simulink model "StateMachine_v3"  (R2015a)
settings: Solver=ode1  StartTime=0.0  StopTime=Inf  FixedStep=0.001  RelTol=1e-3
PreLoadFcn:
  | LoadVar
PostLoadFcn:
  | , if any(exist('dsrtsu_mdlpostloadfcn', 'file') == [2, 3, 6]), try dsrtsu_mdlpostloadfcn('Execute', bdroot); catch fprintf('Error in PostLoadFcn (dsrtsu_mdlpostloadfcn) for model "%s":\n %s\n', bdroot, lasterr); end, end,
values from neighbouring files (symbols this model uses):
  AllowReset = 0    [LoadVar.m]
  Brake_Limits = [Brake_lowerlim1,Brake_upperlim1,Brake_lowerlim2,Brake_upperlim2]    [LoadVar.m]
  DcCLimGen = 0    [LoadVar.m]
  DcCLimMot = 20    [LoadVar.m]
  DcVLimGen = 400    [LoadVar.m]
  DcVLimMot = 280    [LoadVar.m]
  DifferentialFactor = 0.5    [LoadVar.m]
  MaxDisplacementSteeringRack = 21.08    [LoadVar.m]
  MaxSteeringAngle = 24.635    [LoadVar.m]
  MechPwrMaxGen = 3000    [LoadVar.m]
  MechPwrMaxMot = 3000    [LoadVar.m]
  PowerLim_W = 3000    [LoadVar.m]
  SpdSlewrate = 1000    [LoadVar.m]
  Steer_Limits = [Steer_lowerlim,Steer_upperlim,Steer_zero]    [LoadVar.m]
  Susp_Limits = [Susp_lowerlim1,Susp_upperlim1,Susp_lowerlim2,Susp_upperlim2,Susp_lowerlim3,Susp_upperlim3,Susp_lowerlim4,Susp_upperlim4]    [LoadVar.m]
  Throttle_Limits = [Throttle_lowerlim1,Throttle_upperlim1,Throttle_lowerlim2,Throttle_upperlim2]    [LoadVar.m]
  TrqSlewrate = 3    [LoadVar.m]
libraries: rtican x25, rti1401lib_adc_type4 x16, rti1401lib_dio_type3 x16, rtilib1401 x1
(part 7 of 7)

== system StateMachine_v3/PRE-PROCESSOR/SteeringAngleCalculation ==
  SteeringAngleTravel_% : Inport
  limits : Inport  Port=2
  1-D Lookup Table : Lookup_n-D  NumberOfTableDimensions=1  BreakpointsForDimension1=[-MaxDisplacementSteeringRack,-20.1,-19.12,-18.14,-17.15,-16.18,-15.2,-14.22,-13.25,-12.27,-11.3,-10.34,-9.38,-8.42,-7.46,-6.51,-5.56,-4.62,-3.69,-2.75,-1.83,-0.91,0,0.91,1.83,2.75,3.69,4.62,5.56,6.51,7.46,8.42,9.38,10.34,11.3,12.27,13.25,14.22,15.2,16.18,17.15,18.14,19.12,20.1,MaxDisplacementSteeringRack]  Table=[-MaxSteeringAngle,-23.33,-22.06,-20.81,-19.59,-18.385,-17.205,-16.035,-14.855,-13.75,-12.63,-11.52,-10.425,-9.34,-8.265,-7.2,-6.145,-5.1,-4.065,-3.035,-2.015,-1.05,0,1.05,2.015,3.035,4.065,5.1,6.145,7.2,8.265,9.34,10.425,11.52,12.63,13.75,14.855,16.035,17.205,18.385,19.59,20.81,22.06,23.33,MaxSteeringAngle]  InternalRulePriority=Speed  RndMeth=Simplest  InputSameDT=on
  Constant : Constant  Value=MaxDisplacementSteeringRack
  MATLAB Function : MATLAB Function  TreatAsAtomicUnit=on
  SteeringAngle_° : Outport
  SteeringAngleSensorError : Outport  Port=2
  wires:
  MATLAB Function/2(e) -> SteeringAngleSensorError/1
  limits/1 -> MATLAB Function/3(limits)
  MATLAB Function/1(SteeringDisplacement) -> 1-D Lookup Table/1  "SteeringDisplacement_mm"
  SteeringAngleTravel_%/1 -> MATLAB Function/1(SteeringAngleTravel)
  1-D Lookup Table/1 -> SteeringAngle_°/1  "SteeringAngle_°"
  Constant/1 -> MATLAB Function/2(MaxDisplacementSteeringRack)

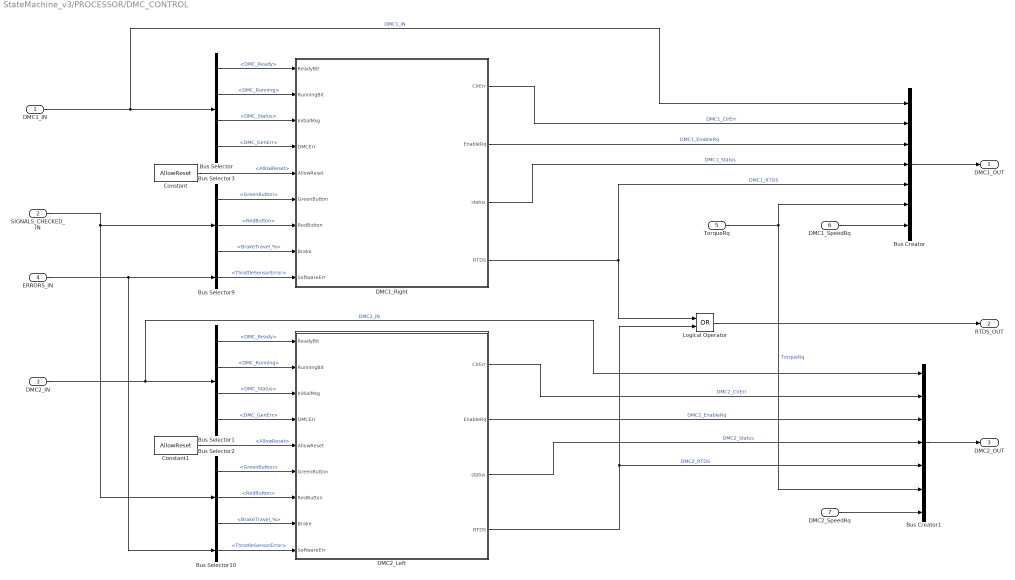
== system StateMachine_v3/PROCESSOR/DMC_CONTROL ==
  DMC1_IN : Inport
  SIGNALS_CHECKED_IN : Inport  Port=2
  DMC2_IN : Inport  Port=3
  ERRORS_IN : Inport  Port=4
  TorqueRq : Inport  Port=5
  DMC1_SpeedRq : Inport  Port=6
  DMC2_SpeedRq : Inport  Port=7
  Bus Creator : BusCreator  Inputs=7
  Bus Creator1 : BusCreator  Inputs=7
  Bus Selector : BusSelector  OutputSignals=DMC_Ready,DMC_Running,DMC_Status,DMC_GenErr
  Bus Selector1 : BusSelector  OutputSignals=DMC_Ready,DMC_Running,DMC_Status,DMC_GenErr
  Bus Selector10 : BusSelector  OutputSignals=ThrottleSensorError
  Bus Selector2 : BusSelector  OutputSignals=SIGNALS.DigitalInputs.GreenButton,SIGNALS.DigitalInputs.RedButton,BrakeTravel_%
  Bus Selector3 : BusSelector  OutputSignals=SIGNALS.DigitalInputs.GreenButton,SIGNALS.DigitalInputs.RedButton,BrakeTravel_%
  Bus Selector9 : BusSelector  OutputSignals=ThrottleSensorError
  Constant : Constant  Value=AllowReset
  Constant1 : Constant  Value=AllowReset
  DMC1_Right : Stateflow chart  TreatAsAtomicUnit=on
  DMC2_Left : Stateflow chart  TreatAsAtomicUnit=on
  Logical Operator : Logic  Operator=OR  AllPortsSameDT=off  OutDataTypeStr=boolean
  DMC1_OUT : Outport
  RTDS_OUT : Outport  Port=2
  DMC2_OUT : Outport  Port=3
  wires:
  TorqueRq/1 -> Bus Creator1/6, Bus Creator/6  "TorqueRq"
  ERRORS_IN/1 -> Bus Selector10/1, Bus Selector9/1
  SIGNALS_CHECKED_IN/1 -> Bus Selector2/1, Bus Selector3/1
  DMC1_Right/3(status) -> Bus Creator/4  "DMC1_Status"
  Bus Creator/1 -> DMC1_OUT/1
  Bus Selector9/1 -> DMC1_Right/9(SoftwareErr)  "<ThrottleSensorError>"
  Bus Selector10/1 -> DMC2_Left/9(SoftwareErr)  "<ThrottleSensorError>"
  Bus Creator1/1 -> DMC2_OUT/1
  Bus Selector/4 -> DMC1_Right/4(DMCErr)  "<DMC_GenErr>"
  Bus Selector3/2 -> DMC1_Right/7(RedButton)  "<RedButton>"
  DMC2_IN/1 -> Bus Creator1/1, Bus Selector1/1  "DMC2_IN"
  Bus Selector1/4 -> DMC2_Left/4(DMCErr)  "<DMC_GenErr>"
  DMC1_SpeedRq/1 -> Bus Creator/7
  DMC2_Left/3(status) -> Bus Creator1/4  "DMC2_Status"
  Bus Selector2/3 -> DMC2_Left/8(Brake)  "<BrakeTravel_%>"
  DMC2_Left/4(RTDS) -> Bus Creator1/5, Logical Operator/2  "DMC2_RTDS"
  DMC1_Right/4(RTDS) -> Logical Operator/1, Bus Creator/5  "DMC1_RTDS"
  Logical Operator/1 -> RTDS_OUT/1
  DMC2_Left/1(ClrErr) -> Bus Creator1/2  "DMC2_ClrErr"
  Constant1/1 -> DMC2_Left/5(AllowReset)  "<AllowReset>"
  Bus Selector1/2 -> DMC2_Left/2(RunningBit)  "<DMC_Running>"
  DMC1_IN/1 -> Bus Creator/1, Bus Selector/1  "DMC1_IN"
  DMC1_Right/1(ClrErr) -> Bus Creator/2  "DMC1_ClrErr"
  DMC2_SpeedRq/1 -> Bus Creator1/7
  Bus Selector1/1 -> DMC2_Left/1(ReadyBit)  "<DMC_Ready>"
  Bus Selector3/1 -> DMC1_Right/6(GreenButton)  "<GreenButton>"
  Bus Selector/3 -> DMC1_Right/3(InitialMsg)  "<DMC_Status>"
  Bus Selector1/3 -> DMC2_Left/3(InitialMsg)  "<DMC_Status>"
  Bus Selector/1 -> DMC1_Right/1(ReadyBit)  "<DMC_Ready>"
  Bus Selector3/3 -> DMC1_Right/8(Brake)  "<BrakeTravel_%>"
  Bus Selector2/2 -> DMC2_Left/7(RedButton)  "<RedButton>"
  DMC2_Left/2(EnableRq) -> Bus Creator1/3  "DMC2_EnableRq"
  Bus Selector/2 -> DMC1_Right/2(RunningBit)  "<DMC_Running>"
  Bus Selector2/1 -> DMC2_Left/6(GreenButton)  "<GreenButton>"
  Constant/1 -> DMC1_Right/5(AllowReset)  "<AllowReset>"
  DMC1_Right/2(EnableRq) -> Bus Creator/3  "DMC1_EnableRq"

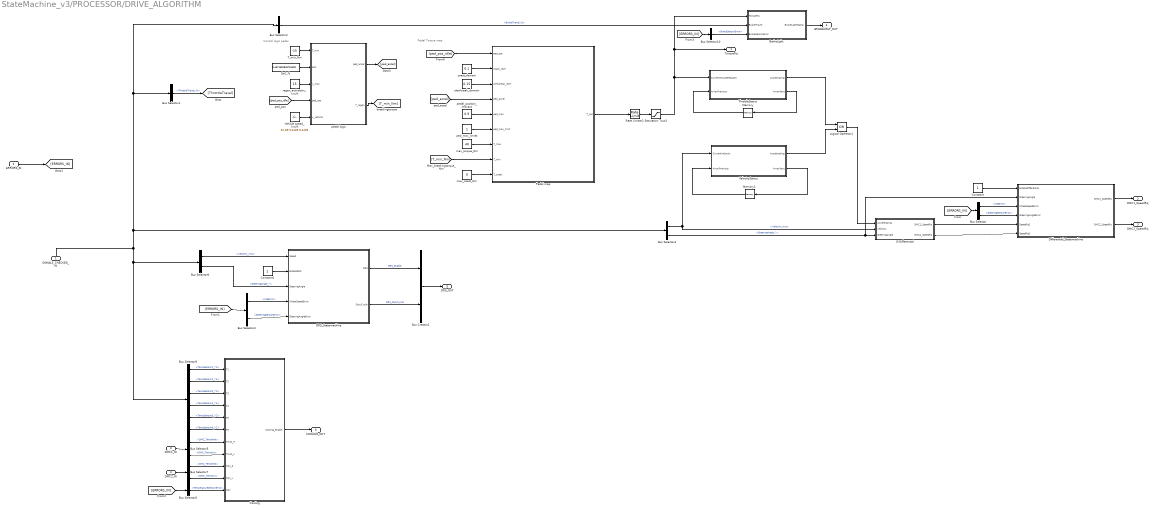
== system StateMachine_v3/PROCESSOR/DRIVE_ALGORITHM ==
  note: Control logic pedal
  note: Pedal Torque map
  SIGNALS_CHECKED_IN : Inport
  ERRORS_IN : Inport  Port=2
  DMC1_IN : Inport  Port=3
  DMC2_IN : Inport  Port=4
  BrakeLight : MATLAB Function  TreatAsAtomicUnit=on
  Bus Creator2 : BusCreator  Inputs=2
  Bus Selector : BusSelector  OutputSignals=WSError,SteeringSensorError
  Bus Selector1 : BusSelector  OutputSignals=ThrottleTravel_%
  Bus Selector10 : BusSelector  OutputSignals=BrakeSensorError
  Bus Selector2 : BusSelector  OutputSignals=BrakeTravel_%
  Bus Selector3 : BusSelector  OutputSignals=WSError,SteeringSensorError
  Bus Selector4 : BusSelector  OutputSignals=Velocity_m/s,SteeringAngle_°
  Bus Selector5 : BusSelector  OutputSignals=DMC_TempMot,DMC_TempInv
  Bus Selector6 : BusSelector  OutputSignals=TemperatureSensorError
  Bus Selector7 : BusSelector  OutputSignals=DMC_TempMot,DMC_TempInv
  Bus Selector8 : BusSelector  OutputSignals=Velocity_m/s,SteeringAngle_°
  Bus Selector9 : BusSelector  OutputSignals=TempSensor1_°C,TempSensor2_°C,TempSensor3_°C,TempSensor4_°C,TempSensor5_°C,TempSensor6_°C
  Constant : Constant
  Constant1 : Constant
  Cooling : MATLAB Function  TreatAsAtomicUnit=on
  DRS_Statemachine : Stateflow chart  TreatAsAtomicUnit=on
  Differential_Statemachine : Stateflow chart  TreatAsAtomicUnit=on
  E-Differential : Subsystem
  Logical Operator1 : Logic  Operator=OR  AllPortsSameDT=off  OutDataTypeStr=boolean
  Memory : Memory  X0=zeros(10,1)  InheritSampleTime=on
  Memory1 : Memory  X0=zeros(10,1)  InheritSampleTime=on
  Pedal map : MATLAB Function  TreatAsAtomicUnit=on
  Rate Limiter2 : RateLimiter  RisingSlewLimit=20  FallingSlewLimit=-20  SampleTimeMode=inherited
  Saturation Tout1 : Saturate  UpperLimit=39  LowerLimit=-39
  SoC_% : Constant  Value=0.4671532846715328
  T_min_Nm : Constant  Value=-15
  ThrottleStatus : MATLAB Function  TreatAsAtomicUnit=on
  Vehicle speed_km/h : Constant  Value=52.85714285714285
  VelocityStatus : MATLAB Function  TreatAsAtomicUnit=on
  coast_domain : Constant  Value=0.1
  max_coast_Nm : Constant  Value=0
  max_torque_Nm : Constant  Value=40
  ped_max_limiet : Constant
  pedal logic : Stateflow chart  TreatAsAtomicUnit=on
  pedal_position_maxacc : Constant  Value=0.9
  regen_activation_km/h : Constant  Value=15
  slewbreak_domain : Constant  Value=0.15
  TorqueRq : Outport
  DMC1_SpeedRq : Outport  Port=2
  DMC2_SpeedRq : Outport  Port=3
  BRAKELIGHT_OUT : Outport  Port=4
  DRS_OUT : Outport  Port=5
  COOLING_OUT : Outport  Port=6
  wires:
  Bus Selector1/1 -> [ThrottleTravel]  "<ThrottleTravel_%>"
  DRS_Statemachine/1(DRS) -> Bus Creator2/1  "DRS_Enable"
  DRS_Statemachine/2(DutyCycle) -> Bus Creator2/2  "DRS_DutyCycle"
  Bus Creator2/1 -> DRS_OUT/1
  Bus Selector8/2 -> DRS_Statemachine/3(SteeringAngle)  "<SteeringAngle_°>"
  Bus Selector8/1 -> DRS_Statemachine/1(Speed)  "<Velocity_m/s>"
  SIGNALS_CHECKED_IN/1 -> Bus Selector1/1, Bus Selector2/1, Bus Selector4/1, Bus Selector9/1, Bus Selector8/1
  Constant1/1 -> DRS_Statemachine/2(EnableDRS)
  Saturation Tout1/1 -> BrakeLight/1(TorqueRq), TorqueRq/1, ThrottleStatus/1(CurrentTorqueRequest)
  Pedal map/1(T_out) -> Rate Limiter2/1
  [ped_accel] -> Pedal map/4(ped_accel)
  Rate Limiter2/1 -> Saturation Tout1/1
  coast_domain/1 -> Pedal map/2(coast_dom)
  Vehicle speed_km/h/1 -> pedal logic/5(v_vehicle)
  [ped_pos_idle] -> pedal logic/4(ped_pos)
  pedal_position_maxacc/1 -> Pedal map/5(ped_max)
  T_min_Nm/1 -> pedal logic/1(T_min)
  ped_max_limiet/1 -> Pedal map/6(ped_max_limit)
  [ped_pos_idle] -> Pedal map/1(ped_pos)
  slewbreak_domain/1 -> Pedal map/3(slewbreak_dom)
  [T_min_Nm] -> Pedal map/8(T_min)
  SoC_%/1 -> pedal logic/2(SoC)
  pedal logic/2(T_regen) -> [T_min_Nm]
  max_torque_Nm/1 -> Pedal map/7(T_max)
  pedal logic/1(ped_accel) -> [ped_accel]
  regen_activation_km/h/1 -> pedal logic/3(v_max)
  max_coast_Nm/1 -> Pedal map/9(T_coast)
  Bus Selector4/2 -> Differential_Statemachine/2(SteeringAngle), E-Differential/3(SteeringAngle)  "<SteeringAngle_°>"
  Bus Selector4/1 -> VelocityStatus/1(CurrentVelocity), E-Differential/2(Velocity)  "<Velocity_m/s>"
  Bus Selector2/1 -> BrakeLight/2(BrakeTravel)  "<BrakeTravel_%>"
  BrakeLight/1(BrakeLightSignal) -> BRAKELIGHT_OUT/1
  Constant/1 -> Differential_Statemachine/1(EnableDifferential)
  Differential_Statemachine/2(DMC2_SpeedRq) -> DMC2_SpeedRq/1
  Differential_Statemachine/1(DMC1_SpeedRq) -> DMC1_SpeedRq/1
  E-Differential/1(DMC1_SpeedRq) -> Differential_Statemachine/5(SpeedRq1)
  E-Differential/2(DMC2_SpeedRq) -> Differential_Statemachine/6(SpeedRq2)
  Memory/1 -> ThrottleStatus/2(ArrayPrevious)
  ThrottleStatus/2(ArrayNext) -> Memory/1
  VelocityStatus/2(ArrayNext) -> Memory1/1
  Memory1/1 -> VelocityStatus/2(ArrayPrevious)
  ThrottleStatus/1(Accelerating) -> Logical Operator1/1
  VelocityStatus/1(Accelerating) -> Logical Operator1/2
  Logical Operator1/1 -> E-Differential/1(Accelerating)
  ERRORS_IN/1 -> [ERRORS_IN]
  [ERRORS_IN] -> Bus Selector/1
  Bus Selector/2 -> Differential_Statemachine/4(SteeringAngleError)  "<SteeringSensorError>"
  Bus Selector/1 -> Differential_Statemachine/3(WheelSpeedError)  "<WSError>"
  Bus Selector3/1 -> DRS_Statemachine/4(WheelSpeedError)  "<WSError>"
  Bus Selector3/2 -> DRS_Statemachine/5(SteeringAngleError)  "<SteeringSensorError>"
  [ERRORS_IN] -> Bus Selector3/1
  DMC1_IN/1 -> Bus Selector5/1
  DMC2_IN/1 -> Bus Selector7/1
  [ERRORS_IN] -> Bus Selector6/1
  Bus Selector9/1 -> Cooling/1(T1)  "<TempSensor1_°C>"
  Bus Selector9/2 -> Cooling/2(T2)  "<TempSensor2_°C>"
  Bus Selector6/1 -> Cooling/11(Terr)  "<TemperatureSensorError>"
  Bus Selector9/4 -> Cooling/4(T4)  "<TempSensor4_°C>"
  Bus Selector9/6 -> Cooling/6(T6)  "<TempSensor6_°C>"
  Bus Selector9/5 -> Cooling/5(T5)  "<TempSensor5_°C>"
  Bus Selector9/3 -> Cooling/3(T3)  "<TempSensor3_°C>"
  Bus Selector5/1 -> Cooling/7(Tmot_R)  "<DMC_TempMot>"
  Bus Selector5/2 -> Cooling/8(Tmot_L)  "<DMC_TempInv>"
  Bus Selector7/1 -> Cooling/9(Tdri_R)  "<DMC_TempMot>"
  Bus Selector7/2 -> Cooling/10(Tdri_L)  "<DMC_TempInv>"
  Cooling/1(Cooling_Enable) -> COOLING_OUT/1
  [ERRORS_IN] -> Bus Selector10/1
  Bus Selector10/1 -> BrakeLight/3(BrakeSensorError)  "<BrakeSensorError>"

== system StateMachine_v3/RTI Data/RTI Data Store ==
  RTI Data Store : Subsystem  mask(RTI_DATA_STORE){}
      mask help:
      | RTI Data Store Block. This block is used by RTI to store internal model dependent data. Deleting this block will result in data loss.
      |
      | NEVER DELETE, COPY, OR MODIFY THIS BLOCK!
      mask Help:
      | RTI Data Store Block. This block is used by RTI to store internal model dependent data. Deleting this block will result in data loss.
      | 
      | NEVER DELETE, COPY, OR MODIFY THIS BLOCK!
      mask Display: text(0.5, 0.5, ' ', 'HorizontalAlignment', 'center');

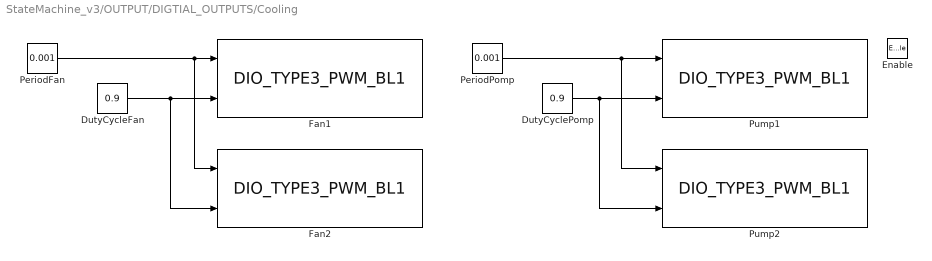
== system StateMachine_v3/OUTPUT/DIGTIAL_OUTPUTS/Cooling ==
  Enable : EnablePort
  DutyCycleFan : Constant  Value=0.9
  DutyCyclePomp : Constant  Value=0.9
  Fan1 : rti1401lib_dio_type3/DIO_TYPE3_PWM_BL1  DSProperties=struct('RTI',struct('Version',uint32(2),'BlockType',struct('isSLSource',uint8(0),'isSLSink',uint8(1),'isHWSource',uint8(0),'isHWSink',uint8(1),'isSetup',uint8(0),'isInline',uint8(1),'isNonInline',uint8(0),'isInterrupt',uint8(0),'isChannelwise',uint8(1)),'IOBoardType',{{'DS1401','STD','DIOT3'}},'UnitType','PWM','Identifier','PWM','DialogType','ML','BlockSet','NONE','SlaveProcessor','NONE'))  RTIBlockInterface=struct('InputPortsWidth',int32([1 1]),'InputPortsActive',[1 1],'InputPortsName',{{'Period',['Duty Cycle']}},'BlockDisplay',{{['DIO TP3 PWM\nModule: 1\nPort: 1\nChannel: 3'],'center'}},'IconTransparency','on','InitLevel',3,'DialogFcn','rti1401stddiot3pwmgui','BlockName',struct('Token',{{'DIO_TYPE3_PWM_BL1'}}))  RTIBlockParameters=struct('ModuleNo',{{1,'OFF',[1 16]}},'PortNo',{{1,'OFF',[1 3]}},'ChannelNo',{{3,'OFF',[1 16]}},'SupplyRailsCh',{{[1 1],'OFF',[0 1 0 1]}},'UpdateMode',{{1,'ON',[1 2]}},'PeriodRange',{{7,'OFF',[1 16]}},'DutyCycleInit',{{'0','OFF',[0 1]}},'PeriodInit',{{'5e-05','OFF',[]}},'TerminationMode',{{0,'OFF',[0 1]}},'OutputTermValidate',{{0,'OFF',[0 1]}},'OutputTermBuildCheck',{{0,'OFF',[]}},'DutyCycleTerm',{{'0','OFF',[0 1]}},'PeriodTerm',{{'5e-05','OFF',[]}},'TLCFileName',{{'rti1401dio_t3_pwm','OFF',[]}},'EnableInterrupt',{{0,'OFF',[0 1]}},'TriggerEdgeType',{{1,'OFF',[1 3]}})  RTISFcnParameters=struct('ModuleNo','int32','PortNo','int16','ChannelNo','int16','SupplyRailsCh','int16','UpdateMode','int16','PeriodRange','int16','DutyCycleInit','double','PeriodInit','double','TerminationMode','int16','OutputTermValidate','int16','DutyCycleTerm','double','PeriodTerm','double','TLCFileName','char','EnableInterrupt','int16','TriggerEdgeType','int32')  RTIBlockParaDefault=struct('ModuleNo',1,'PortNo',1,'ChannelNo',1,'SupplyRailsCh',[1 1],'UpdateMode',1,'PeriodRange',7,'DutyCycleInit',0,'PeriodInit',5e-05,'TerminationMode',0,'OutputTermValidate',0,'OutputTermBuildCheck',0,'DutyCycleTerm',0,'PeriodTerm',5e-05,'TLCFileName','rti1401dio_t3_pwm','EnableInterrupt',0,'TriggerEdgeType',1)
  Fan2 : rti1401lib_dio_type3/DIO_TYPE3_PWM_BL1  DSProperties=struct('RTI',struct('Version',uint32(2),'BlockType',struct('isSLSource',uint8(0),'isSLSink',uint8(1),'isHWSource',uint8(0),'isHWSink',uint8(1),'isSetup',uint8(0),'isInline',uint8(1),'isNonInline',uint8(0),'isInterrupt',uint8(0),'isChannelwise',uint8(1)),'IOBoardType',{{'DS1401','STD','DIOT3'}},'UnitType','PWM','Identifier','PWM','DialogType','ML','BlockSet','NONE','SlaveProcessor','NONE'))  RTIBlockInterface=struct('InputPortsWidth',int32([1 1]),'InputPortsActive',[1 1],'InputPortsName',{{'Period',['Duty Cycle']}},'BlockDisplay',{{['DIO TP3 PWM\nModule: 1\nPort: 1\nChannel: 4'],'center'}},'IconTransparency','on','InitLevel',3,'DialogFcn','rti1401stddiot3pwmgui','BlockName',struct('Token',{{'DIO_TYPE3_PWM_BL1'}}))  RTIBlockParameters=struct('ModuleNo',{{1,'OFF',[1 16]}},'PortNo',{{1,'OFF',[1 3]}},'ChannelNo',{{4,'OFF',[1 16]}},'SupplyRailsCh',{{[1 1],'OFF',[0 1 0 1]}},'UpdateMode',{{1,'ON',[1 2]}},'PeriodRange',{{7,'OFF',[1 16]}},'DutyCycleInit',{{'0','OFF',[0 1]}},'PeriodInit',{{'5e-05','OFF',[]}},'TerminationMode',{{0,'OFF',[0 1]}},'OutputTermValidate',{{0,'OFF',[0 1]}},'OutputTermBuildCheck',{{0,'OFF',[]}},'DutyCycleTerm',{{'0','OFF',[0 1]}},'PeriodTerm',{{'5e-05','OFF',[]}},'TLCFileName',{{'rti1401dio_t3_pwm','OFF',[]}},'EnableInterrupt',{{0,'OFF',[0 1]}},'TriggerEdgeType',{{1,'OFF',[1 3]}})  RTISFcnParameters=struct('ModuleNo','int32','PortNo','int16','ChannelNo','int16','SupplyRailsCh','int16','UpdateMode','int16','PeriodRange','int16','DutyCycleInit','double','PeriodInit','double','TerminationMode','int16','OutputTermValidate','int16','DutyCycleTerm','double','PeriodTerm','double','TLCFileName','char','EnableInterrupt','int16','TriggerEdgeType','int32')  RTIBlockParaDefault=struct('ModuleNo',1,'PortNo',1,'ChannelNo',1,'SupplyRailsCh',[1 1],'UpdateMode',1,'PeriodRange',7,'DutyCycleInit',0,'PeriodInit',5e-05,'TerminationMode',0,'OutputTermValidate',0,'OutputTermBuildCheck',0,'DutyCycleTerm',0,'PeriodTerm',5e-05,'TLCFileName','rti1401dio_t3_pwm','EnableInterrupt',0,'TriggerEdgeType',1)
  PeriodFan : Constant  Value=0.001
  PeriodPomp : Constant  Value=0.001
  Pump1 : rti1401lib_dio_type3/DIO_TYPE3_PWM_BL1  DSProperties=struct('RTI',struct('Version',uint32(2),'BlockType',struct('isSLSource',uint8(0),'isSLSink',uint8(1),'isHWSource',uint8(0),'isHWSink',uint8(1),'isSetup',uint8(0),'isInline',uint8(1),'isNonInline',uint8(0),'isInterrupt',uint8(0),'isChannelwise',uint8(1)),'IOBoardType',{{'DS1401','STD','DIOT3'}},'UnitType','PWM','Identifier','PWM','DialogType','ML','BlockSet','NONE','SlaveProcessor','NONE'))  RTIBlockInterface=struct('InputPortsWidth',int32([1 1]),'InputPortsActive',[1 1],'InputPortsName',{{'Period',['Duty Cycle']}},'BlockDisplay',{{['DIO TP3 PWM\nModule: 1\nPort: 1\nChannel: 5'],'center'}},'IconTransparency','on','InitLevel',3,'DialogFcn','rti1401stddiot3pwmgui','BlockName',struct('Token',{{'DIO_TYPE3_PWM_BL1'}}))  RTIBlockParameters=struct('ModuleNo',{{1,'OFF',[1 16]}},'PortNo',{{1,'OFF',[1 3]}},'ChannelNo',{{5,'OFF',[1 16]}},'SupplyRailsCh',{{[1 1],'OFF',[0 1 0 1]}},'UpdateMode',{{1,'ON',[1 2]}},'PeriodRange',{{7,'OFF',[1 16]}},'DutyCycleInit',{{'0','OFF',[0 1]}},'PeriodInit',{{'5e-05','OFF',[]}},'TerminationMode',{{0,'OFF',[0 1]}},'OutputTermValidate',{{0,'OFF',[0 1]}},'OutputTermBuildCheck',{{0,'OFF',[]}},'DutyCycleTerm',{{'0','OFF',[0 1]}},'PeriodTerm',{{'5e-05','OFF',[]}},'TLCFileName',{{'rti1401dio_t3_pwm','OFF',[]}},'EnableInterrupt',{{0,'OFF',[0 1]}},'TriggerEdgeType',{{1,'OFF',[1 3]}})  RTISFcnParameters=struct('ModuleNo','int32','PortNo','int16','ChannelNo','int16','SupplyRailsCh','int16','UpdateMode','int16','PeriodRange','int16','DutyCycleInit','double','PeriodInit','double','TerminationMode','int16','OutputTermValidate','int16','DutyCycleTerm','double','PeriodTerm','double','TLCFileName','char','EnableInterrupt','int16','TriggerEdgeType','int32')  RTIBlockParaDefault=struct('ModuleNo',1,'PortNo',1,'ChannelNo',1,'SupplyRailsCh',[1 1],'UpdateMode',1,'PeriodRange',7,'DutyCycleInit',0,'PeriodInit',5e-05,'TerminationMode',0,'OutputTermValidate',0,'OutputTermBuildCheck',0,'DutyCycleTerm',0,'PeriodTerm',5e-05,'TLCFileName','rti1401dio_t3_pwm','EnableInterrupt',0,'TriggerEdgeType',1)
  Pump2 : rti1401lib_dio_type3/DIO_TYPE3_PWM_BL1  DSProperties=struct('RTI',struct('Version',uint32(2),'BlockType',struct('isSLSource',uint8(0),'isSLSink',uint8(1),'isHWSource',uint8(0),'isHWSink',uint8(1),'isSetup',uint8(0),'isInline',uint8(1),'isNonInline',uint8(0),'isInterrupt',uint8(0),'isChannelwise',uint8(1)),'IOBoardType',{{'DS1401','STD','DIOT3'}},'UnitType','PWM','Identifier','PWM','DialogType','ML','BlockSet','NONE','SlaveProcessor','NONE'))  RTIBlockInterface=struct('InputPortsWidth',int32([1 1]),'InputPortsActive',[1 1],'InputPortsName',{{'Period',['Duty Cycle']}},'BlockDisplay',{{['DIO TP3 PWM\nModule: 1\nPort: 1\nChannel: 6'],'center'}},'IconTransparency','on','InitLevel',3,'DialogFcn','rti1401stddiot3pwmgui','BlockName',struct('Token',{{'DIO_TYPE3_PWM_BL1'}}))  RTIBlockParameters=struct('ModuleNo',{{1,'OFF',[1 16]}},'PortNo',{{1,'OFF',[1 3]}},'ChannelNo',{{6,'OFF',[1 16]}},'SupplyRailsCh',{{[1 1],'OFF',[0 1 0 1]}},'UpdateMode',{{1,'ON',[1 2]}},'PeriodRange',{{7,'OFF',[1 16]}},'DutyCycleInit',{{'0','OFF',[0 1]}},'PeriodInit',{{'5e-05','OFF',[]}},'TerminationMode',{{0,'OFF',[0 1]}},'OutputTermValidate',{{0,'OFF',[0 1]}},'OutputTermBuildCheck',{{0,'OFF',[]}},'DutyCycleTerm',{{'0','OFF',[0 1]}},'PeriodTerm',{{'5e-05','OFF',[]}},'TLCFileName',{{'rti1401dio_t3_pwm','OFF',[]}},'EnableInterrupt',{{0,'OFF',[0 1]}},'TriggerEdgeType',{{1,'OFF',[1 3]}})  RTISFcnParameters=struct('ModuleNo','int32','PortNo','int16','ChannelNo','int16','SupplyRailsCh','int16','UpdateMode','int16','PeriodRange','int16','DutyCycleInit','double','PeriodInit','double','TerminationMode','int16','OutputTermValidate','int16','DutyCycleTerm','double','PeriodTerm','double','TLCFileName','char','EnableInterrupt','int16','TriggerEdgeType','int32')  RTIBlockParaDefault=struct('ModuleNo',1,'PortNo',1,'ChannelNo',1,'SupplyRailsCh',[1 1],'UpdateMode',1,'PeriodRange',7,'DutyCycleInit',0,'PeriodInit',5e-05,'TerminationMode',0,'OutputTermValidate',0,'OutputTermBuildCheck',0,'DutyCycleTerm',0,'PeriodTerm',5e-05,'TLCFileName','rti1401dio_t3_pwm','EnableInterrupt',0,'TriggerEdgeType',1)
  wires:
  DutyCyclePomp/1 -> Pump2/2, Pump1/2
  DutyCycleFan/1 -> Fan2/2, Fan1/2
  PeriodPomp/1 -> Pump2/1, Pump1/1
  PeriodFan/1 -> Fan2/1, Fan1/1

== system StateMachine_v3/OUTPUT/DIGTIAL_OUTPUTS/DRS ==
  ServoFrequency : Inport
  Enable : EnablePort
  Divide : Product  Inputs=*/
  Gain : Gain  Gain=0.000001
  PWM DRS : rti1401lib_dio_type3/DIO_TYPE3_PWM_BL1  DSProperties=struct('RTI',struct('Version',uint32(2),'BlockType',struct('isSLSource',uint8(0),'isSLSink',uint8(1),'isHWSource',uint8(0),'isHWSink',uint8(1),'isSetup',uint8(0),'isInline',uint8(1),'isNonInline',uint8(0),'isInterrupt',uint8(0),'isChannelwise',uint8(1)),'IOBoardType',{{'DS1401','STD','DIOT3'}},'UnitType','PWM','Identifier','PWM','DialogType','ML','BlockSet','NONE','SlaveProcessor','NONE'))  RTIBlockInterface=struct('InputPortsWidth',int32([1 1]),'InputPortsActive',[1 1],'InputPortsName',{{'Period',['Duty Cycle']}},'BlockDisplay',{{['DIO TP3 PWM\nModule: 1\nPort: 1\nChannel: 7'],'center'}},'IconTransparency','on','InitLevel',3,'DialogFcn','rti1401stddiot3pwmgui','BlockName',struct('Token',{{'DIO_TYPE3_PWM_BL1'}}))  RTIBlockParameters=struct('ModuleNo',{{1,'OFF',[1 16]}},'PortNo',{{1,'OFF',[1 3]}},'ChannelNo',{{7,'OFF',[1 16]}},'SupplyRailsCh',{{[1 1],'OFF',[0 1 0 1]}},'UpdateMode',{{1,'ON',[1 2]}},'PeriodRange',{{7,'OFF',[1 16]}},'DutyCycleInit',{{'0','OFF',[0 1]}},'PeriodInit',{{'5e-05','OFF',[]}},'TerminationMode',{{0,'OFF',[0 1]}},'OutputTermValidate',{{0,'OFF',[0 1]}},'OutputTermBuildCheck',{{0,'OFF',[]}},'DutyCycleTerm',{{'0','OFF',[0 1]}},'PeriodTerm',{{'5e-05','OFF',[]}},'TLCFileName',{{'rti1401dio_t3_pwm','OFF',[]}},'EnableInterrupt',{{0,'OFF',[0 1]}},'TriggerEdgeType',{{1,'OFF',[1 3]}})  RTISFcnParameters=struct('ModuleNo','int32','PortNo','int16','ChannelNo','int16','SupplyRailsCh','int16','UpdateMode','int16','PeriodRange','int16','DutyCycleInit','double','PeriodInit','double','TerminationMode','int16','OutputTermValidate','int16','DutyCycleTerm','double','PeriodTerm','double','TLCFileName','char','EnableInterrupt','int16','TriggerEdgeType','int32')  RTIBlockParaDefault=struct('ModuleNo',1,'PortNo',1,'ChannelNo',1,'SupplyRailsCh',[1 1],'UpdateMode',1,'PeriodRange',7,'DutyCycleInit',0,'PeriodInit',5e-05,'TerminationMode',0,'OutputTermValidate',0,'OutputTermBuildCheck',0,'DutyCycleTerm',0,'PeriodTerm',5e-05,'TLCFileName','rti1401dio_t3_pwm','EnableInterrupt',0,'TriggerEdgeType',1)
  PWM DRS1 : rti1401lib_dio_type3/DIO_TYPE3_PWM_BL1  DSProperties=struct('RTI',struct('Version',uint32(2),'BlockType',struct('isSLSource',uint8(0),'isSLSink',uint8(1),'isHWSource',uint8(0),'isHWSink',uint8(1),'isSetup',uint8(0),'isInline',uint8(1),'isNonInline',uint8(0),'isInterrupt',uint8(0),'isChannelwise',uint8(1)),'IOBoardType',{{'DS1401','STD','DIOT3'}},'UnitType','PWM','Identifier','PWM','DialogType','ML','BlockSet','NONE','SlaveProcessor','NONE'))  RTIBlockInterface=struct('InputPortsWidth',int32([1 1]),'InputPortsActive',[1 1],'InputPortsName',{{'Period',['Duty Cycle']}},'BlockDisplay',{{['DIO TP3 PWM\nModule: 1\nPort: 1\nChannel: 8'],'center'}},'IconTransparency','on','InitLevel',3,'DialogFcn','rti1401stddiot3pwmgui','BlockName',struct('Token',{{'DIO_TYPE3_PWM_BL1'}}))  RTIBlockParameters=struct('ModuleNo',{{1,'OFF',[1 16]}},'PortNo',{{1,'OFF',[1 3]}},'ChannelNo',{{8,'OFF',[1 16]}},'SupplyRailsCh',{{[1 1],'OFF',[0 1 0 1]}},'UpdateMode',{{1,'ON',[1 2]}},'PeriodRange',{{7,'OFF',[1 16]}},'DutyCycleInit',{{'0','OFF',[0 1]}},'PeriodInit',{{'5e-05','OFF',[]}},'TerminationMode',{{0,'OFF',[0 1]}},'OutputTermValidate',{{0,'OFF',[0 1]}},'OutputTermBuildCheck',{{0,'OFF',[]}},'DutyCycleTerm',{{'0','OFF',[0 1]}},'PeriodTerm',{{'5e-05','OFF',[]}},'TLCFileName',{{'rti1401dio_t3_pwm','OFF',[]}},'EnableInterrupt',{{0,'OFF',[0 1]}},'TriggerEdgeType',{{1,'OFF',[1 3]}})  RTISFcnParameters=struct('ModuleNo','int32','PortNo','int16','ChannelNo','int16','SupplyRailsCh','int16','UpdateMode','int16','PeriodRange','int16','DutyCycleInit','double','PeriodInit','double','TerminationMode','int16','OutputTermValidate','int16','DutyCycleTerm','double','PeriodTerm','double','TLCFileName','char','EnableInterrupt','int16','TriggerEdgeType','int32')  RTIBlockParaDefault=struct('ModuleNo',1,'PortNo',1,'ChannelNo',1,'SupplyRailsCh',[1 1],'UpdateMode',1,'PeriodRange',7,'DutyCycleInit',0,'PeriodInit',5e-05,'TerminationMode',0,'OutputTermValidate',0,'OutputTermBuildCheck',0,'DutyCycleTerm',0,'PeriodTerm',5e-05,'TLCFileName','rti1401dio_t3_pwm','EnableInterrupt',0,'TriggerEdgeType',1)
  PeriodDRS : Constant  Value=0.008
  wires:
  PeriodDRS/1 -> Divide/2, PWM DRS1/1, PWM DRS/1
  ServoFrequency/1 -> Gain/1
  Divide/1 -> PWM DRS1/2, PWM DRS/2
  Gain/1 -> Divide/1

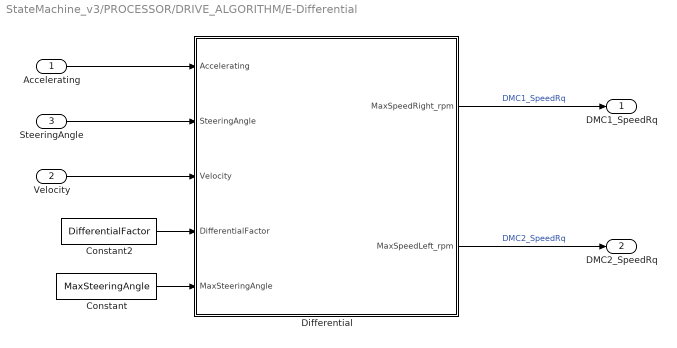
== system StateMachine_v3/PROCESSOR/DRIVE_ALGORITHM/E-Differential ==
  Accelerating : Inport
  Velocity : Inport  Port=2
  SteeringAngle : Inport  Port=3
  Constant : Constant  Value=MaxSteeringAngle
  Constant2 : Constant  Value=DifferentialFactor
  Differential : MATLAB Function  TreatAsAtomicUnit=on
  DMC1_SpeedRq : Outport
  DMC2_SpeedRq : Outport  Port=2
  wires:
  SteeringAngle/1 -> Differential/2(SteeringAngle)
  Velocity/1 -> Differential/3(Velocity)
  Constant2/1 -> Differential/4(DifferentialFactor)
  Differential/2(MaxSpeedLeft_rpm) -> DMC2_SpeedRq/1  "DMC2_SpeedRq"
  Differential/1(MaxSpeedRight_rpm) -> DMC1_SpeedRq/1  "DMC1_SpeedRq"
  Accelerating/1 -> Differential/1(Accelerating)
  Constant/1 -> Differential/5(MaxSteeringAngle)

== system StateMachine_v3/RTI Data/RTI Data Store/RTI Data Store ==
  RTI Data Store : Subsystem  mask(RTI_DATA_STORE){}
      mask help:
      | RTI Data Store Block. This block is used by RTI to store internal model dependent data. Deleting this block will result in data loss.
      |
      | NEVER DELETE, COPY, OR MODIFY THIS BLOCK!
      mask Help:
      | RTI Data Store Block. This block is used by RTI to store internal model dependent data. Deleting this block will result in data loss.
      | 
      | NEVER DELETE, COPY, OR MODIFY THIS BLOCK!
      mask Display: text(0.5, 0.5, ' ', 'HorizontalAlignment', 'center');

== system StateMachine_v3/RTI Data/RTI Data Store/RTI Data Store/RTI Data Store ==
  RTI Data Store : Subsystem  mask(RTI_DATA_STORE){}
      mask help:
      | RTI Data Store Block. This block is used by RTI to store internal model dependent data. Deleting this block will result in data loss.
      |
      | NEVER DELETE, COPY, OR MODIFY THIS BLOCK!
      mask Help:
      | RTI Data Store Block. This block is used by RTI to store internal model dependent data. Deleting this block will result in data loss.
      | 
      | NEVER DELETE, COPY, OR MODIFY THIS BLOCK!
      mask Display: text(0.5, 0.5, ' ', 'HorizontalAlignment', 'center');

== system StateMachine_v3/RTI Data/RTI Data Store/RTI Data Store/RTI Data Store/RTI Data Store ==

== stateflow chart StateMachine_v3/PROCESSOR/DMC_CONTROL/DMC1_Right ==
  note: dSpace en DMC krijgen stroom doordat LV switch wordt omgedraaid
  state CheckCAN
    entry: status = 0;
    entry: EnableRq = 0;
    entry: ClrErr = 0;
    entry: RTDS = 0;
  note: Juiste bericht wordt opgesteld en voor de eerste keer verzonden door de dSpace
      | DMC zendt voor de eerste keer zijn berichten
  note: dSpace kijkt of hoe alle CAN berichten voor de eerste keer heeft ontvangen
  state InitialErrorClearing
    entry: status = 1;
    entry: EnableRq = 0;
    entry: ClrErr = 1;
  note: Alle berichten eens ontvangen, dus error clearen door van 0 -> 1 te zetten
  state Error
    entry: status = 2;
    entry: EnableRq = 0;
    entry: ClrErr = 0;
    entry: RTDS = 0;
  note: Conditie dat beide AIRs zijn gesloten
  note: Conditie dat beide AIRs zijn gesloten
  state ErrorFreeFrame
    state Offline
      entry: status = 4;
      entry: EnableRq = 0;
    state TimerOn
    state TimerOff
    state InitialisationRTD
      entry: status = 5;
      entry: EnableRq = 1;
      entry: ClrErr = 0;
      entry: RTDS = 1;
    state RTD
      entry: status = 6;
      entry: EnableRq = 1;
      entry: RTDS = 0;
    TimerOff -> Offline [order 2] : after(1,sec)
    Offline -> TimerOn : [ReadyBit == 1 && GreenButton == 1 && Brake > 50]
    TimerOn -> Offline [order 2] : [GreenButton == 0 || Brake < 50]
    TimerOn -> InitialisationRTD [order 1] : after (2,sec)
    TimerOff -> RTD [order 1] : [RedButton == 0]
    RTD -> TimerOff : [RedButton == 1]
    InitialisationRTD -> RTD : [RunningBit == 1 && after(2,sec)]
  state Reset
    entry: status = 3;
    entry: EnableRq = 0;
    entry: ClrErr = 1;
  (default) -> CheckCAN
  CheckCAN -> InitialErrorClearing : [InitialMsg == 1]
  InitialErrorClearing -> Error : [after(1,sec)]
  ErrorFreeFrame -> Error : [DMCErr == 1 || SoftwareErr == 1]
  Error -> Reset [order 2] : [AllowReset == 1 && (DMCErr == 1 || SoftwareErr == 1)]
  Error -> Offline [order 1] : [DMCErr == 0 && SoftwareErr ==0]
  Reset -> Offline
  data: ClrErr output; ReadyBit input; RunningBit input; InitialMsg input; DMCErr input; AllowReset input; GreenButton input; RedButton input; Brake input; EnableRq output; status output; RTDS output; SoftwareErr input

== matlab function StateMachine_v3/PRE-PROCESSOR/TemperatureConverter ==
  data: Vin input; u1 input; u2 input; u3 input; u4 input; u5 input; u6 input; y1 output; y2 output; y3 output; y4 output; y5 output; y6 output; e1 output; e2 output; e3 output; e4 output; e5 output; e6 output
function [y1,y2,y3,y4,y5,y6,e1,e2,e3,e4,e5,e6] = TemperatureConverter(Vin,u1,u2,u3,u4,u5,u6)

% Calculation in °C
y1 = 3435/(log((u1*0.1)/(Vin-u1))+11.521046)-273.15;
y2 = 3435/(log((u2*0.1)/(Vin-u2))+11.521046)-273.15;
y3 = 3435/(log((u3*0.1)/(Vin-u3))+11.521046)-273.15;
y4 = 3435/(log((u4*0.1)/(Vin-u4))+11.521046)-273.15;
y5 = 3435/(log((u5*0.1)/(Vin-u5))+11.521046)-273.15;
y6 = 3435/(log((u5*0.1)/(Vin-u6))+11.521046)-273.15;

% Errors
if y1 > 200 || y1 < 0
    e1 = 0;
else
    e1 = 1;
end
if y2 > 200 || y2 < 0
    e2 = 0;
else
    e2 = 1;
end
if y3 > 200 || y3 < 0
    e3 = 0;
else
    e3 = 1;
end
if y4 > 200 || y4 < 0
    e4 = 0;
else
    e4 = 1;
end
if y5 > 200 || y5 < 0
    e5 = 0;
else
    e5 = 1;
end
if y6 > 200 || y6 < 0
    e6 = 0;
else
    e6 = 1;
end

== stateflow chart StateMachine_v3/PROCESSOR/DMC_CONTROL/DMC2_Left ==
  note: dSpace en DMC krijgen stroom doordat LV switch wordt omgedraaid
  state CheckCAN
    entry: status = 0;
    entry: EnableRq = 0;
    entry: ClrErr = 0;
    entry: RTDS = 0;
  note: Juiste bericht wordt opgesteld en voor de eerste keer verzonden door de dSpace
      | DMC zendt voor de eerste keer zijn berichten
  note: dSpace kijkt of hoe alle CAN berichten voor de eerste keer heeft ontvangen
  state InitialErrorClearing
    entry: status = 1;
    entry: EnableRq = 0;
    entry: ClrErr = 1;
  note: Alle berichten eens ontvangen, dus error clearen door van 0 -> 1 te zetten
  state Error
    entry: status = 2;
    entry: EnableRq = 0;
    entry: ClrErr = 0;
    entry: RTDS = 0;
  note: Conditie dat beide AIRs zijn gesloten
  note: Conditie dat beide AIRs zijn gesloten
  state Reset
    entry: status = 3;
    entry: EnableRq = 0;
    entry: ClrErr = 1;
  state ErrorFreeFrame
    state Offline
      entry: status = 4;
      entry: EnableRq = 0;
    state TimerOn
    state TimerOff
    state InitialisationRTD
      entry: status = 5;
      entry: EnableRq = 1;
      entry: ClrErr = 0;
      entry: RTDS = 1;
    state RTD
      entry: status = 6;
      entry: EnableRq = 1;
      entry: RTDS = 0;
    TimerOff -> Offline [order 2] : after(1,sec)
    Offline -> TimerOn : [ReadyBit == 1 && GreenButton == 1 && Brake > 50]
    TimerOn -> Offline [order 2] : [GreenButton == 0 || Brake < 50]
    TimerOn -> InitialisationRTD [order 1] : after (2,sec)
    RTD -> TimerOff : [RedButton == 1]
    TimerOff -> RTD [order 1] : [RedButton == 0]
    InitialisationRTD -> RTD : [RunningBit == 1 && after(2,sec)]
  (default) -> CheckCAN
  CheckCAN -> InitialErrorClearing : [InitialMsg == 1]
  InitialErrorClearing -> Error : [after(1,sec)]
  ErrorFreeFrame -> Error : [DMCErr == 1 || SoftwareErr == 1]
  Error -> Reset [order 2] : [AllowReset == 1 && (DMCErr == 1 || SoftwareErr == 1)]
  Error -> Offline [order 1] : [DMCErr == 0 && SoftwareErr == 0]
  Reset -> Offline
  data: ClrErr output; ReadyBit input; RunningBit input; InitialMsg input; DMCErr input; AllowReset input; GreenButton input; RedButton input; Brake input; EnableRq output; status output; RTDS output; SoftwareErr input

== matlab function StateMachine_v3/PROCESSOR/DRIVE_ALGORITHM/BrakeLight ==
  data: TorqueRq input; BrakeTravel input; BrakeLightSignal output; BrakeSensorError input
function BrakeLightSignal = BrakeLight(TorqueRq,BrakeTravel, BrakeSensorError)

if BrakeTravel > 0 || TorqueRq < 0 && BrakeSensorError == 0
    BrakeLightSignal = true;
else
    BrakeLightSignal = false;
end

== matlab function StateMachine_v3/PROCESSOR/DRIVE_ALGORITHM/ThrottleStatus ==
  data: CurrentTorqueRequest input; ArrayPrevious input; Accelerating output; ArrayNext output
function [Accelerating, ArrayNext] = MovingAverage(CurrentTorqueRequest, ArrayPrevious)
% Calculates the moving average of the matrix defined in the memory block

% Calculation of moving average
TorqueAverage = mean(ArrayPrevious);
ArrayNext = circshift(ArrayPrevious,1);
ArrayNext(1) = CurrentTorqueRequest;

% Looks whether the current torque request exceeds the mean of the previous 100ms torque commands
if CurrentTorqueRequest > TorqueAverage && CurrentTorqueRequest > 0
    Accelerating = 1;
else
    Accelerating = 0;
end

== matlab function StateMachine_v3/PRE-PROCESSOR/SteeringAngleCalculation/MATLAB Function ==
  data: SteeringAngleTravel input; MaxDisplacementSteeringRack input; SteeringDisplacement output; limits input; e output
function [SteeringDisplacement, e] = SteeringConverter(SteeringAngleTravel, MaxDisplacementSteeringRack, limits)
% Positive SteeringDisplacement is used for a right corner

% Variables
lowerlim = limits(1);
upperlim = limits(2);
zerolim = limits(3);

% SteeringSensor
if SteeringAngleTravel < lowerlim
    SteeringDisplacement = -MaxDisplacementSteeringRack;
elseif SteeringAngleTravel > upperlim
    SteeringDisplacement = MaxDisplacementSteeringRack;   
elseif SteeringAngleTravel == zerolim
    SteeringDisplacement = 0;
elseif SteeringAngleTravel > zerolim
    SteeringDisplacement =(MaxDisplacementSteeringRack/(upperlim-zerolim))*(SteeringAngleTravel-zerolim);
else
    SteeringDisplacement = ((-MaxDisplacementSteeringRack/(zerolim-lowerlim))*(SteeringAngleTravel-lowerlim)+MaxDisplacementSteeringRack)*-1;   
end


% ErrorCheck
if SteeringAngleTravel < 0.10 || SteeringAngleTravel > 0.90   
    e = 1;
else
    e = 0;
end

== matlab function StateMachine_v3/PRE-PROCESSOR/WSConverter ==
  data: WS_FR input; WS_FR_rpm output; WS_FL input; WS_RR input; WS_RL input; WS_FL_rpm output; WS_RR_rpm output; WS_RL_rpm output; Velocity_mps output; LongitudinalSlip output; e output
function [WS_FR_rpm, WS_FL_rpm, WS_RR_rpm, WS_RL_rpm, Velocity_mps, LongitudinalSlip, e] = WSConverter(WS_FR, WS_FL, WS_RR, WS_RL)

% Calculation
NumberOfPulses = 46;
TireRadius = 0.4572/2;

WS_FR_rpm = WS_FR/NumberOfPulses*60;
WS_FL_rpm = WS_FL/NumberOfPulses*60;
WS_RR_rpm = WS_RR/NumberOfPulses*60;
WS_RL_rpm = WS_RL/NumberOfPulses*60;

WS_FR_mps = WS_FR_rpm*2*pi/60*TireRadius;
WS_FL_mps = WS_FL_rpm*2*pi/60*TireRadius;
WS_RR_mps = WS_RR_rpm*2*pi/60*TireRadius;
WS_RL_mps = WS_RL_rpm*2*pi/60*TireRadius;

% Error plausible result
if WS_FR_rpm < -50 || WS_FR_rpm > 18000
    e_FR = 1;
else
    e_FR = 0;
    WS_FR_rpm = 0;
end
if WS_FL_rpm < -50 || WS_FL_rpm > 18000
    e_FL = 1;
else
    e_FL = 0;
    WS_FL_rpm = 0;
end
if WS_RR_rpm < -50 || WS_RR_rpm > 18000
    e_RR = 1;
else
    e_RR = 0;
    WS_RR_rpm = 0;
end
if WS_RL_rpm < -50 || WS_RL_rpm > 18000
    e_RL = 1;
else
    e_RL = 0;
    WS_RL_rpm = 0;
end

% Correct action
if e_FR == 0 && e_FL == 0
    
    Velocity_mps = (WS_FR_mps + WS_FL_mps)/2;
    e = 0;
    if e_RR == 0 && e_RL == 0
        LongitudinalSlip = ((WS_RR_mps + WS_RL_mps)/2- Velocity_mps)/Velocity_mps;
    else
        LongitudinalSlip = 0;
    end
    
elseif e_FR == 0 && e_FL == 1   
    
    Velocity_mps = WS_FR_mps;
    e =0;
    if e_RR == 0 && e_RL == 0
        LongitudinalSlip = ((WS_RR_mps + WS_RL_mps)/2- Velocity_mps)/Velocity_mps;
    else
        LongitudinalSlip = 0;
    end
    
elseif e_FR == 1 && e_FL == 0
    
    Velocity_mps = WS_FL_mps;
    e = 0;
    if e_RR == 0 && e_RL == 0
        LongitudinalSlip = ((WS_RR_mps + WS_RL_mps)/2- Velocity_mps)/Velocity_mps;
    else
        LongitudinalSlip = 0;
    end   
    
else
    e = 1;
    Velocity_mps = 0;
    LongitudinalSlip = 0;
   
end

== matlab function StateMachine_v3/PROCESSOR/DRIVE_ALGORITHM/Pedal map ==
  data: ped_pos input; coast_dom input; T_out output; slewbreak_dom input; ped_accel input; ped_max input; ped_max_limit input; T_max input; T_min input; T_coast input
function T_out = Pedalmap_eq(ped_pos,coast_dom,slewbreak_dom,ped_accel,ped_max,ped_max_limit,T_max,T_min,T_coast)
%%Accelerator pedal mapping:

ped_regen=ped_accel-coast_dom; %pedal postion - start regen - variable in function of velocity
ped_zero=ped_regen-slewbreak_dom; %pedal postion - start max regen - variable in function of velocity

slewrate_acc=(T_max-T_coast)/(ped_max-ped_accel); %slewrate acceleration region
slewrate_regen=(T_min-T_coast)/(ped_zero-ped_regen);%slewrate regen region

% acceleration pedal map eq.
T_out=T_min*(heavi(ped_pos,0)-heavi(ped_pos,ped_zero)) + (slewrate_regen*(ped_pos-ped_regen)+T_coast)*(heavi(ped_pos,ped_zero)-heavi(ped_pos,ped_regen))+T_coast*(heavi(ped_pos,ped_regen)-heavi(ped_pos,ped_accel))+(slewrate_acc*(ped_pos-ped_accel)+T_coast)*(heavi(ped_pos,ped_accel)-heavi(ped_pos,ped_max))+T_max*(heavi(ped_pos,ped_max-heavi(ped_pos,ped_max_limit)));

== matlab function StateMachine_v3/PRE-PROCESSOR/ThrottleSensorCalcuation ==
  data: e2 output; e1 output; u1 input; u2 input; y output; limits input
function [e2,e1,y] = ThrottleSensorCalculation(u1, u2, limits)

% Variables
lowerlim1 = limits(1);
upperlim1 = limits(2);
lowerlim2 = limits(3);
upperlim2 = limits(4);

% ThrottleSensor1
t1 = 1-u1;
if t1 < lowerlim1
    y1 = 0;
elseif t1 > upperlim1
    y1 = 1;   
else
    y1 = (1/(upperlim1-lowerlim1))*(t1-lowerlim1);
end

% ThrottleSensor2
t2 = (1-u2);
if t2 < lowerlim2
    y2 = 0;
elseif t2 > upperlim2
    y2 = 1;   
else
    y2 = (1/(upperlim2-lowerlim2))*(t2-lowerlim2);
end

% ErrorCheck
if u1 > 0.10 && u1 < 0.90 && u2 > 0.10 && u2 < 0.90   
    if abs(y1-y2) > 0.10
        e1 = 1;
        e2 = 1;
        y = 0;
    else
        e1 = 0;
        e2 = 0;
        y = (y1+y2)/2;
    end
else
    if (u1 < 0.10 || u1 > 0.90) && (u2 < 0.10 || u2 > 0.90)
        e1 = 1;
        e2 = 1;
        y = 0;
    elseif u1 < 0.10 || u1 > 0.90
        e1 = 1;
        e2 = 0;
        y = y2;
    else
        e1 = 0;
        e2 = 1;
        y = y1;
    end  
    
%     e1 = 1;
%     e2 = 1;
%     y = 0;
end

== matlab function StateMachine_v3/PRE-PROCESSOR/BrakeSensorCalculation ==
  data: y output; u1 input; u2 input; e1 output; e2 output; limits input
function [y,e1,e2] = BrakeSensorCalculation(u1, u2,limits)

% Variables
lowerlim1 = limits(1);
upperlim1 = limits(2);
lowerlim2 = limits(3);
upperlim2 = limits(4);

% BrakeeSensor1
t1 = (1-u1);
if t1 < lowerlim1
    y1 = 0;
elseif t1 > upperlim1
    y1 = 1;   
else
    y1 = (1/(upperlim1-lowerlim1))*(t1-lowerlim1);
end

% BrakeSensor2
t2 = (1-u2);
if t2 < lowerlim2
    y2 = 0;
elseif t2 > upperlim2
    y2 = 1;   
else
    y2 = (1/(upperlim2-lowerlim2))*(t2-lowerlim2);
end

% ErrorCheck
if u1 > 0.10 && u1 < 0.90 && u2 > 0.10 && u2 < 0.90   
    if abs(y1-y2) > 0.10
        e1 = 1;
        e2 = 1;
        y = 0;
    else
        e1 = 0;
        e2 = 0;
        y = (y1+y2)/2;
    end
else
    
    
    if (u1 < 0.10 || u1 > 0.90) && (u2 < 0.10 || u2 > 0.90)
        e1 = 1;
        e2 = 1;
        y = 0;
    elseif u1 < 0.10 || u1 > 0.90
        e1 = 1;
        e2 = 0;
        y = y2;
    else
        e1 = 0;
        e2 = 1;
        y = y1;
    end  
    
%     e1 = 1;
%     e2 = 1;
%     y = 0;
end

== stateflow chart StateMachine_v3/PROCESSOR/DRIVE_ALGORITHM/DRS_Statemachine ==
  state Offline
    entry: DRS = 0;
  state Dicht
    entry:
    DRS = 1;
    DutyCycle = 2100;
  state Open
    entry:
    DRS = 1;
    DutyCycle = 1000;
  (default) -> Offline
  Open -> Offline [order 2] : [EnableDRS == 0]
  Dicht -> Offline [order 1] : [EnableDRS == 0]
  Offline -> Dicht : [EnableDRS == 1]
  Open -> Dicht [order 1] : [Speed < 10 || abs(SteeringAngle) < 5  || WheelSpeedError == 1 || SteeringAngleError == 1]
  Dicht -> Open [order 2] : [Speed > 15 && abs(SteeringAngle) > 10 && WheelSpeedError == 0 && SteeringAngleError == 0]
  data: Speed input; EnableDRS input; DRS output; DutyCycle output; SteeringAngle input; WheelSpeedError input; SteeringAngleError input

== stateflow chart StateMachine_v3/PROCESSOR/DRIVE_ALGORITHM/pedal logic ==
  state Driving
    state Disable_regen %SoC is to high.
      entry:
      ped_accel=0.45;
      T_regen=0;
    state Activate_regen
      entry:
      ped_accel=0.45;
      T0= -5; %Regentorque at v_max [Nm]
      during:
      % velocity dependant braking torque
      if v_vehicle<15
      T_regen=T_min/15
      elseif v_vehicle<50
      T_regen=T_min
      else
      T_regen=(T_min-T0)/(50-100)*(v_vehicle-100)+T0
      end
    (default) -> Disable_regen %SoC is to high.
    Disable_regen %SoC is to high. -> Activate_regen : [SoC<0.95]
    Activate_regen -> Disable_regen %SoC is to high. : [SoC>0.95]
  state Standstill
    entry:
    T_regen=0;
    ped_accel=0.1; %
    during:
    %velocity dependent coasting until v_max
    if ped_pos>0.1
    ped_accel=min(ped_pos* (v_vehicle/v_max),0.45); %Offset of 0.1
    end
    exit:
    ped_accel=0.45;
  (default) -> Standstill
  Driving -> Standstill : [v_vehicle<=5]
  Standstill -> Driving : [v_vehicle >v_max&&ped_pos>0.45]
  data: T_min input; SoC input; v_max input; ped_pos input; v_vehicle input; ped_accel output; T_regen output; T0 local

== matlab function StateMachine_v3/PRE-PROCESSOR/MATLAB Function1 ==
  data: PowerLim_W input; CurrentPower input; ArrayPrevious input; PowerAverage_W output; PowerWarning output; PowerError output; ArrayNext output
function [PowerAverage_W, PowerWarning, PowerError, ArrayNext] = MovingAverage(PowerLim_W, CurrentPower, ArrayPrevious)
% Calculates the moving average of the matrix defined in the memory block

% Calculation of moving average
ArrayNext = circshift(ArrayPrevious,1);
ArrayNext(1) = CurrentPower;
PowerAverage_W = mean(ArrayNext);

% Warning function that warns if a 300ms moving average or a 50ms continuous has exceeded the 80 kW limit
WarningArray_500ms = ArrayNext(1:30);
WarningArray_100ms = ArrayNext(1:5);
if mean(WarningArray_500ms) >= PowerLim_W || min(WarningArray_100ms) >= PowerLim_W
    PowerWarning = 1;
else
    PowerWarning = 0;
end

% Error function that states a 500ms moving average or the 100ms continuous has exceeded the 80 kW limit
ErrorArray_100ms = ArrayNext(1:10);
if PowerAverage_W > PowerLim_W || min(ErrorArray_100ms) >= PowerLim_W
    PowerError = 1;
else
    PowerError = 0;
end

== stateflow chart StateMachine_v3/PROCESSOR/DRIVE_ALGORITHM/Differential_Statemachine ==
  state Offline
    entry:
    DMC1_SpeedRq = 14000;
    DMC2_SpeedRq = 14000;
  state Standby
    entry:
    DMC1_SpeedRq = 14000;
    DMC2_SpeedRq = 14000;
  state Online
    entry:
    DMC1_SpeedRq = SpeedRq1;
    DMC2_SpeedRq = SpeedRq2;
  (default) -> Offline
  (junction 28) -> Offline : [EnableDifferential == 0 || SteeringAngleError == 1 || WheelSpeedError == 1]
  Offline -> Standby : [EnableDifferential == 1 && SteeringAngleError == 0 && WheelSpeedError == 0]
  Standby -> (junction 28) [order 2]
  Online -> (junction 28) [order 2]
  Online -> Standby [order 1] : [abs(SteeringAngle) < 3]
  Standby -> Online [order 1] : [abs(SteeringAngle) > 2]
  data: EnableDifferential input; SteeringAngle input; WheelSpeedError input; SteeringAngleError input; SpeedRq1 input; SpeedRq2 input; DMC1_SpeedRq output; DMC2_SpeedRq output

== matlab function StateMachine_v3/PROCESSOR/DRIVE_ALGORITHM/E-Differential/Differential ==
  data: Accelerating input; MaxSpeedRight_rpm output; MaxSpeedLeft_rpm output; SteeringAngle input; Velocity input; DifferentialFactor input; MaxSteeringAngle input
function [MaxSpeedRight_rpm,MaxSpeedLeft_rpm] = Differential(Accelerating,SteeringAngle, Velocity, DifferentialFactor,MaxSteeringAngle)
% Positive Turn = Right Turn
% Negative Turn = Left Turn

TrackWidth = 1.200; % d in m
TrackLength = 1.534; % L in m
GearRatio = 10.364; % i
TireRadius = 0.4572/2; % r in m

TurnRadius =  TrackLength/tan(SteeringAngle*pi/180); % R in m
TurnSpeed = Velocity/TurnRadius; % Omega in rad/s
if Accelerating == 1
    MaxSpeedRight_mps = (TurnRadius - TrackWidth/2)*TurnSpeed + DifferentialFactor*(MaxSteeringAngle-abs(SteeringAngle))/MaxSteeringAngle; % V_r in m/s
    MaxSpeedLeft_mps = (TurnRadius + TrackWidth/2)*TurnSpeed + DifferentialFactor*(MaxSteeringAngle-abs(SteeringAngle))/MaxSteeringAngle; % V_l in m/s        
else
  	MaxSpeedRight_mps = (TurnRadius - TrackWidth/2)*TurnSpeed;
    MaxSpeedLeft_mps = (TurnRadius + TrackWidth/2)*TurnSpeed;
end
MaxSpeedRight_rpm = MaxSpeedRight_mps/TireRadius*60/2/pi*GearRatio; % V_r in rpm
MaxSpeedLeft_rpm = MaxSpeedLeft_mps/TireRadius*60/2/pi*GearRatio; % V_l in rpm

== matlab function StateMachine_v3/PROCESSOR/DRIVE_ALGORITHM/VelocityStatus ==
  data: CurrentVelocity input; ArrayPrevious input; Accelerating output; ArrayNext output
function [Accelerating, ArrayNext] = MovingAverage(CurrentVelocity, ArrayPrevious)
% Calculates the moving average of the matrix defined in the memory block

% Calculation of moving average
VelocityAverage = mean(ArrayPrevious);
ArrayNext = circshift(ArrayPrevious,1);
ArrayNext(1) = CurrentVelocity;

% Looks whether the current torque request exceeds the mean of the previous 100ms torque commands
if CurrentVelocity > VelocityAverage && CurrentVelocity > 0
    Accelerating = 1;
else
    Accelerating = 0;
end

== matlab function StateMachine_v3/PRE-PROCESSOR/LinearSensorCalculation ==
  data: y1 output; y2 output; y3 output; y4 output; e1 output; e2 output; u1 input; u2 input; u3 input; u4 input; e3 output; limits input; e4 output
function [y1,y2,y3,y4,e1,e2,e3,e4] = LinearSensorCalculation(u1, u2, u3, u4, limits)

lowerlim1 = limits(1);
upperlim1 = limits(2);
lowerlim2 = limits(3);
upperlim2 = limits(4);
lowerlim3 = limits(5);
upperlim3 = limits(6);
lowerlim4 = limits(7);
upperlim4 = limits(8);

% LinearSensor1
if u1 < lowerlim1
    y1 = 0;
elseif u1 > upperlim1
    y1 = 1;   
else
    y1 = (1/(upperlim1-lowerlim1))*(u1-lowerlim1);
end

% LinearSensor2
if u2 < lowerlim2
    y2 = 0;
elseif u2 > upperlim2
    y2 = 1;   
else
    y2 = (1/(upperlim2-lowerlim2))*(u2-lowerlim2);
end

% LinearSensor3
if u3 < lowerlim3
    y3 = 0;
elseif u3 > upperlim3
    y3 = 1;   
else
    y3 = (1/(upperlim3-lowerlim3))*(u3-lowerlim3);
end

% LinearSensor4
if u4 < lowerlim4
    y4 = 0;
elseif u4 > upperlim4
    y4 = 1;   
else
    y4 = (1/(upperlim4-lowerlim4))*(u4-lowerlim4);
end


% ErrorCheck
if u1 < 0.10 || u1 > 0.90   
    e1 = 0;
else
    e1 = 1;
end
if u2 < 0.10 || u2 > 0.90   
    e2 = 0;
else
    e2 = 1;
end
if u3 < 0.10 || u3 > 0.90   
    e3 = 0;
else
    e3 = 1;
end
if u4 < 0.10 || u4 > 0.90   
    e4 = 0;
else
    e4 = 1;
end

== matlab function StateMachine_v3/PROCESSOR/DRIVE_ALGORITHM/Cooling ==
  data: T1 input; Cooling_Enable output; T2 input; T3 input; T4 input; T5 input; T6 input; Tmot_R input; Tmot_L input; Tdri_R input; Tdri_L input; Terr input
function Cooling_Enable = Cooling(T1,T2,T3,T4,T5,T6,Tmot_R,Tmot_L,Tdri_R,Tdri_L,Terr)
% Determines whether the cooling needs to be turned on or off

if Terr == 1 || T1 > 25 || T2 > 25 || T3 > 25 || T4 > 25 || T5 > 25 || T6 > 25 || Tmot_R > 50 || Tmot_L > 50 || Tdri_R > 40 || Tdri_L > 40
    Cooling_Enable = 1;
else
    Cooling_Enable = 0;
end
